simulink model "helicopter_hat"  (R2021b)
settings: Solver=VariableStepAuto  StartTime=0.0  StopTime=T  RelTol=1e-4
values from neighbouring files (symbols this model uses):
  b = 0    [FI_observable.m]
undefined symbols (not defined in the file or in its folder): K1, K3, K4
settings Model: Creator=lcaric  LastModifiedBy=lcaric
settings SolverCC: AlgebraicLoopSolver=TrustRegion
settings DataIOCC: ReturnWorkspaceOutputs=off
settings DebuggingCC: SFMachineParentedDataDiag=warning  ArithmeticOperatorsInVariantConditions=warning
settings SFSimCC: CustomCodeUndefinedFunction=UseInterfaceOnly

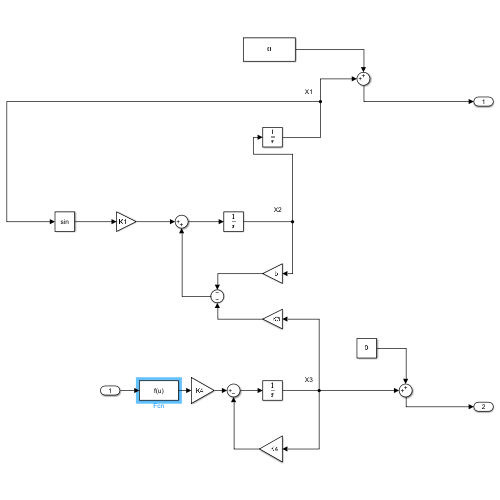
[thumbnail: Simulink's stored preview of the top-level diagram]
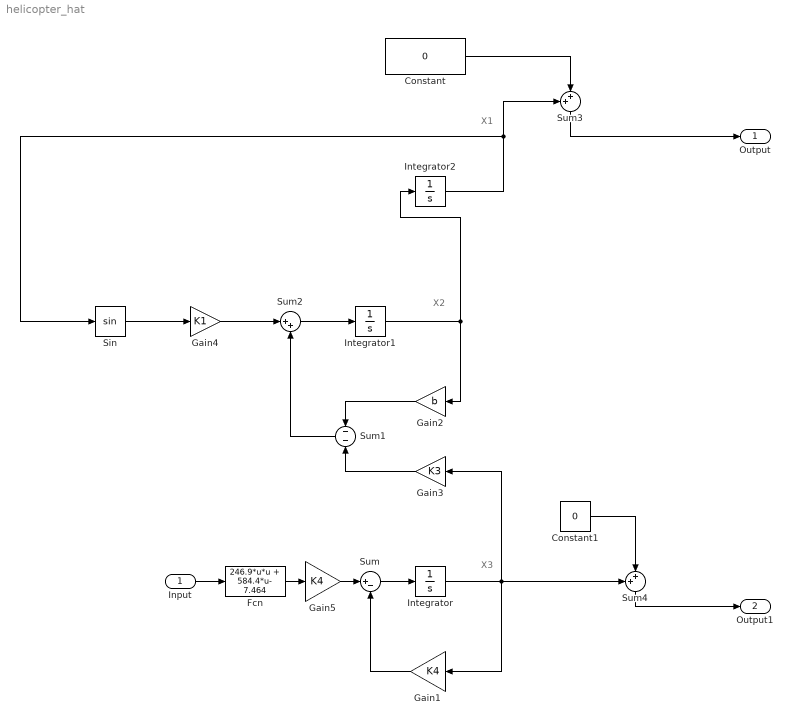
== system helicopter_hat ==
  note: X1
  note: X2
  note: X3
  Input : Inport
  Constant : Constant  Value=0
  Constant1 : Constant  Value=0
  Fcn : Fcn  Expr=246.9*u*u + 584.4*u- 7.464
  Gain1 : Gain  Gain=K4
  Gain2 : Gain  Gain=b
  Gain3 : Gain  Gain=K3
  Gain4 : Gain  Gain=K1
  Gain5 : Gain  Gain=K4
  Integrator : Integrator
  Integrator1 : Integrator  AbsoluteTolerance=10e-4
  Integrator2 : Integrator
  Sin : Trigonometry
  Sum : Sum  Inputs=|+-
  Sum1 : Sum  Inputs=--
  Sum2 : Sum  Inputs=|++
  Sum3 : Sum  Inputs=++|
  Sum4 : Sum  Inputs=++|
  Output : Outport  VectorParamsAs1DForOutWhenUnconnected=off
  Output1 : Outport  Port=2  VectorParamsAs1DForOutWhenUnconnected=off
  wires:
  Gain1/1 -> Sum/2
  Sum/1 -> Integrator/1
  Integrator/1 -> Sum4/1, Gain3/1, Gain1/1
  Gain2/1 -> Sum1/1
  Gain3/1 -> Sum1/2
  Integrator2/1 -> Sum3/1, Sin/1
  Sum1/1 -> Sum2/2
  Sin/1 -> Gain4/1
  Sum2/1 -> Integrator1/1
  Gain4/1 -> Sum2/1
  Input/1 -> Fcn/1
  Integrator1/1 -> Gain2/1, Integrator2/1
  Sum3/1 -> Output/1
  Constant/1 -> Sum3/2
  Sum4/1 -> Output1/1
  Constant1/1 -> Sum4/2
  Fcn/1 -> Gain5/1
  Gain5/1 -> Sum/1
